simulink model "Model_ParachuteJump_14b"  (R2014b)
settings: Solver=ode45  StartTime=0.0  StopTime=10.0  RelTol=1e-3
undefined symbols (not defined in the file or in its folder): in
settings Model: Creator=Arek  LastModifiedBy=Arek
settings SolverCC: ZeroCrossAlgorithm=Adaptive

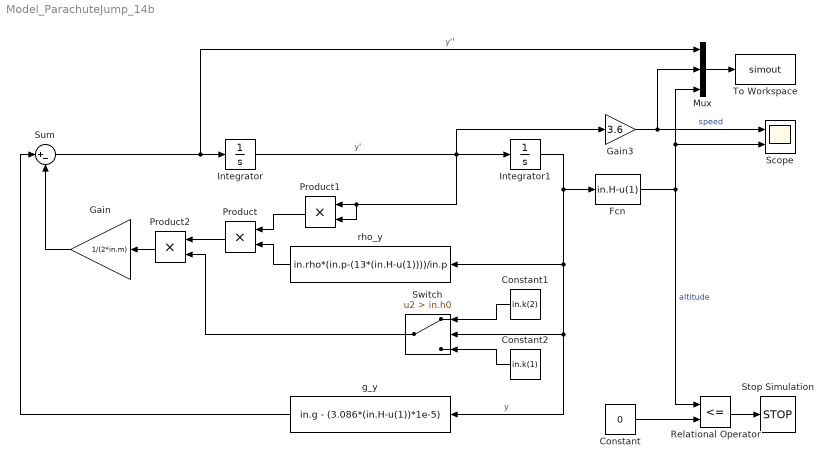
== system Model_ParachuteJump_14b ==
  Constant : Constant  Value=0
  Constant1 : Constant  Value=in.k(2)
  Constant2 : Constant  Value=in.k(1)
  Fcn : Fcn  Expr=in.H-u(1)
  Gain : Gain  Gain=1/(2*in.m)
  Gain3 : Gain  Gain=3.6
  Integrator : Integrator
  Integrator1 : Integrator
  Mux : Mux  Inputs=3
  Product : Product
  Product1 : Product
  Product2 : Product
  Relational Operator : RelationalOperator  Operator=<=  OutDataTypeStr=boolean
  Scope : Scope  NumInputPorts=2
      settings: ShowLegends=on  YMin=-5~-5  YMax=5~5
  Stop Simulation : Stop
  Sum : Sum  Inputs=|+-
  Switch : Switch  Criteria=u2 > Threshold  Threshold=in.h0
  To Workspace : ToWorkspace  VariableName=simout  SaveFormat=Timeseries  SampleTime=-1
  g_y : Fcn  Expr=in.g - (3.086*(in.H-u(1))*1e-5)
  rho_y : Fcn  Expr=in.rho*(in.p-(13*(in.H-u(1))))/in.p
  wires:
  Integrator/1 -> Gain3/1, Product1/2, Product1/1, Integrator1/1  "y'"
  Integrator1/1 -> g_y/1, Switch/2, rho_y/1, Fcn/1  "y"
  Sum/1 -> Mux/1, Integrator/1  "y''"
  Gain/1 -> Sum/2
  g_y/1 -> Sum/1
  Mux/1 -> To Workspace/1
  rho_y/1 -> Product/2
  Fcn/1 -> Mux/3, Scope/2, Relational Operator/1  "altitude"
  Relational Operator/1 -> Stop Simulation/1
  Constant/1 -> Relational Operator/2
  Gain3/1 -> Scope/1, Mux/2  "speed"
  Product1/1 -> Product/1
  Product2/1 -> Gain/1
  Product/1 -> Product2/1
  Switch/1 -> Product2/2
  Constant1/1 -> Switch/1
  Constant2/1 -> Switch/3
